simulink model "goal_example"  (R2025b)
settings: Solver=VariableStepAuto  StartTime=0.0  StopTime=1  RelTol=1e-3
libraries: ros2lib x3
settings Model: Creator=kjhaydon  LastModifiedBy=kjhaydon

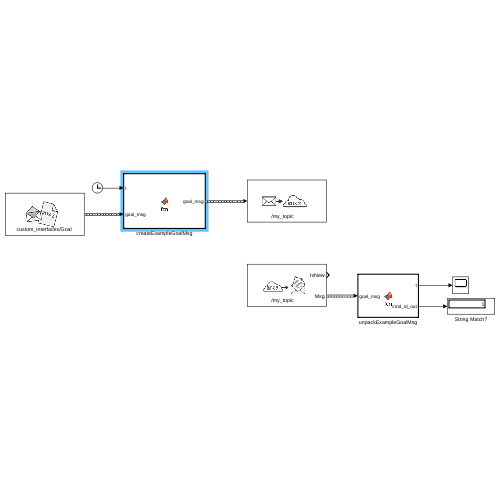
[thumbnail: Simulink's stored preview of the top-level diagram]
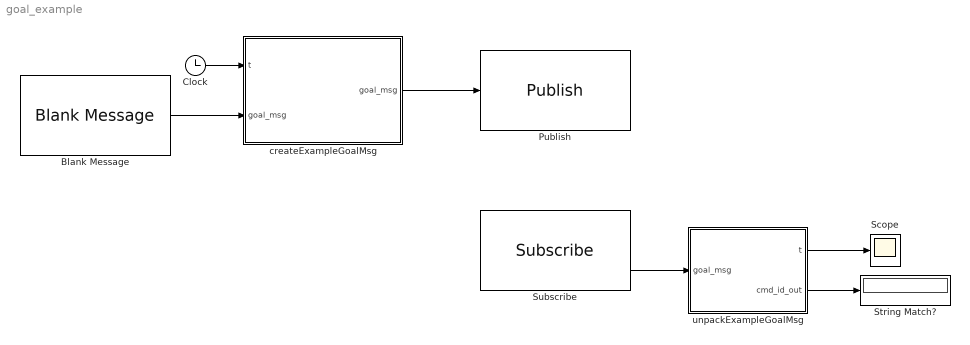
== system goal_example ==
  Blank Message : ros2lib/Blank Message  messageClass=Message  entityType=custom_interfaces/Goal  messageType=custom_interfaces/Goal  SampleTime=0.01
  Clock : Clock
  Publish : ros2lib/Publish  topicSource=Specify your own  topic=/my_topic  messageType=custom_interfaces/Goal  QOSHistory=Keep last  QOSDepth=10  QOSReliability=Reliable  QOSDurability=Volatile  QOSDeadline=Inf  QOSLifespan=Inf  QOSLiveliness=Automatic  QOSLeaseDuration=Inf  QOSAvoidROSNamespaceConventions=off
  Scope : Scope
      settings: ActiveDisplayYMinimum=-1  ActiveDisplayYMaximum=1
  String Match? : Display
  Subscribe : ros2lib/Subscribe  topicSource=Specify your own  topic=/my_topic  messageType=custom_interfaces/Goal  sampleTime=0.01  QOSHistory=Keep last  QOSDepth=10  QOSReliability=Reliable  QOSDurability=Volatile  QOSDeadline=Inf  QOSLifespan=Inf  QOSLiveliness=Automatic  QOSLeaseDuration=Inf  QOSAvoidROSNamespaceConventions=off
  createExampleGoalMsg : MATLAB Function  TreatAsAtomicUnit=on
  unpackExampleGoalMsg : MATLAB Function  TreatAsAtomicUnit=on
  wires:
  Clock/1 -> createExampleGoalMsg/1(t)
  createExampleGoalMsg/1(goal_msg) -> Publish/1
  Blank Message/1 -> createExampleGoalMsg/2("goal_msg ")
  unpackExampleGoalMsg/1(t) -> Scope/1
  Subscribe/2 -> unpackExampleGoalMsg/1(goal_msg)
  unpackExampleGoalMsg/2(cmd_id_out) -> String Match?/1

== matlab function goal_example/createExampleGoalMsg ==
  data: t input; goal_msg output; goal_msg input Bus: SL_Bus_custom_interfaces_Goal
function goal_msg = fcn(t, goal_msg)

%{
Creates a Goal message and populates it with dummy values for testing. For
debugging purposes, the simulation time t is used for goal_msg.waypoint.x.
%}

% Primitive fields
%{
By default Matlab turns strings into 128 element long vectors of uint8_t.
This means we need to pad any strings we are putting into the message to
the same length.
%}


goal_msg.command_id = toFixedLengthUInt("example_cmd");
goal_msg.hold_time  = 1.0; 
goal_msg.object     = toFixedLengthUInt("example_obj");
goal_msg.confidence = 1.0;
goal_msg.trick      = toFixedLengthUInt("example_trick");
goal_msg.duration   = 1.0;

% Nested: Pose6D waypoint (floats)
goal_msg.waypoint.x     = t;
goal_msg.waypoint.y     = 1.0;
goal_msg.waypoint.z     = 1.0;
goal_msg.waypoint.roll  = 1.0;
goal_msg.waypoint.pitch = 1.0;
goal_msg.waypoint.yaw   = 1.0;

% Nested: WaypointMask waypoint_mask (booleans)
goal_msg.waypoint_mask.x     = true;
goal_msg.waypoint_mask.y     = true;
goal_msg.waypoint_mask.z     = false;
goal_msg.waypoint_mask.roll  = false;
goal_msg.waypoint_mask.pitch = false;
goal_msg.waypoint_mask.yaw   = true;

% Nested: Pose6D tolerance (floats)
goal_msg.tolerance.x     = 0.1;
goal_msg.tolerance.y     = 0.1;
goal_msg.tolerance.z     = 0.1;
goal_msg.tolerance.roll  = 0.05;
goal_msg.tolerance.pitch = 0.05;
goal_msg.tolerance.yaw   = 0.05;

end

function output = toFixedLengthUInt(input)
%{
Helper function that inputs a string and outputs a [16x1] vector of char.
If the input is less than 16 characters it is padded with underscores. If
the input is greater than 16 characters, it is trimmed to length.
%}
    input = char(input);        % ensure char array (handles string type too)
    n = length(input);

    if n >= 16
        output = input(1:16);   % trim
    else
        output = [input, repmat('_', 1, 16 - n)];   % pad
    end

    output = uint8(output)';
end

== matlab function goal_example/unpackExampleGoalMsg ==
  data: goal_msg input Bus: SL_Bus_custom_interfaces_Goal; t output; cmd_id_out output
function [t, cmd_id_out] = fcn(goal_msg)

%{
Unpack the field from goal_msg containing t from createExampleGoalMsg.
%}

t = goal_msg.waypoint.x;

%An example of parsing string fields
command_id = goal_msg.command_id;
command_id_char = char(command_id');

%Compare with a switch
switch command_id_char
    case toFixedLengthChar("example_cmd")
        cmd_id_out = 1.0;
    otherwise
        cmd_id_out = 0.0;
end

end



function output = toFixedLengthChar(input)
%{
Helper function that inputs a string and outputs a [1x16] vector of char.
If the input is less than 16 characters it is padded with underscores. If
the input is greater than 16 characters, it is trimmed to length.
%}
    input = char(input);        % ensure char array (handles string type too)
    n = length(input);

    if n >= 16
        output = input(1:16);   % trim
    else
        output = [input, repmat('_', 1, 16 - n)];   % pad
    end

end
